simulink model "SrmUnlineSplineMat7a4b"  (R2014a)
settings: Solver=ode45  StartTime=0.0  StopTime=2  MaxStep=5e-5  RelTol=1e-3
InitFcn:
  | Res=1.5
  | L_0=0.001;
libraries: powerlib x26
settings Model: Creator=Administrator  LastModifiedBy=Think127
settings DataIOCC: SignalLoggingSaveFormat=ModelDataLogs
settings OptimizationCC: ExpressionDepthLimit=2147483647
settings DebuggingCC: UnderspecifiedInitializationDetection=Classic  FcnCallInpInsideContextMsg=UseLocalSettings  StateNameClashWarn=warning
settings GRTTargetCC: CombineOutputUpdateFcns=off  GRTInterface=on

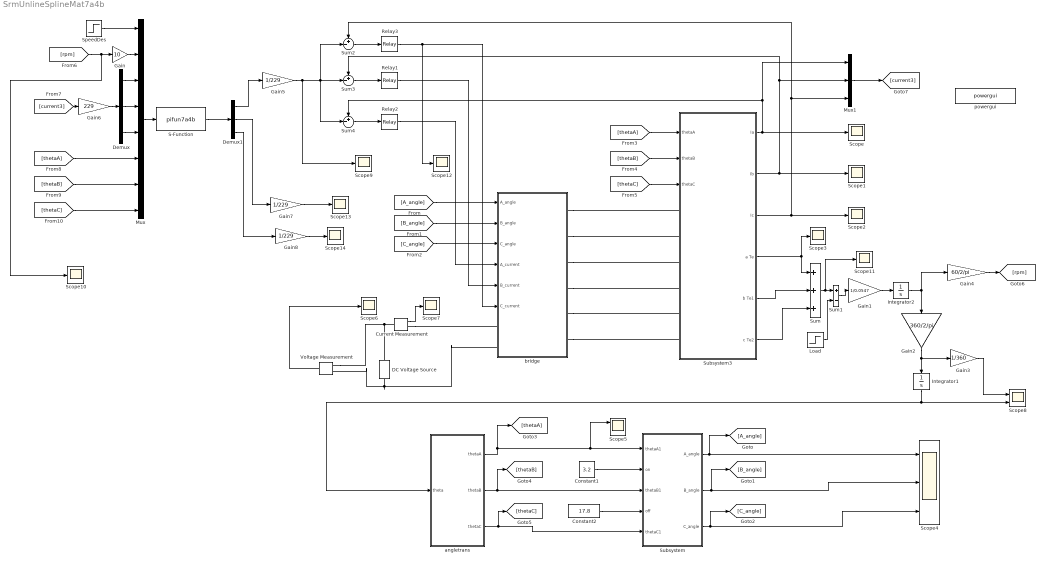
== system SrmUnlineSplineMat7a4b ==
  Constant1 : Constant  Value=3.2
  Constant2 : Constant  Value=17.8
  Current Measurement : powerlib/Measurements/Current Measurement  PhasorSimulation=off  OutputType=Complex  PSBequivalent=0
  DC Voltage Source : powerlib/Electrical Sources/DC Voltage Source  Amplitude=500  Measurements=None
  Demux : Demux  Outputs=3
  Demux1 : Demux  Outputs=3
  Gain : Gain  Gain=10
  Gain1 : Gain  Gain=1/0.0547
  Gain2 : Gain  Gain=360/2/pi
  Gain3 : Gain  Gain=1/360
  Gain4 : Gain  Gain=60/2/pi
  Gain5 : Gain  Gain=1/229
  Gain6 : Gain  Gain=229
  Gain7 : Gain  Gain=1/229
  Gain8 : Gain  Gain=1/229
  Integrator1 : Integrator  InitialCondition=6.5
  Integrator2 : Integrator
  Load : Step  Time=0.3  Before=10  After=10  SampleTime=0
  Mux : Mux  Inputs=8
  Mux1 : Mux  Inputs=3
  Relay1 : Relay  OnSwitchValue=0.1  OffSwitchValue=-0.001  OnOutputValue=0  OffOutputValue=1
  Relay2 : Relay  OnSwitchValue=0.1  OffSwitchValue=-0.001  OnOutputValue=0  OffOutputValue=1
  Relay3 : Relay  OnSwitchValue=0.1  OffSwitchValue=-0.001  OnOutputValue=0  OffOutputValue=1
  S-Function : S-Function  FunctionName=pifun7a4b  EnableBusSupport=off
  Scope{,1..3,6..7,9..14} (12 alike) : Scope
      Scope settings: TimeRange=2  YMin=0  YMax=2.75  SaveName=ScopeDataia
      Scope1 settings: TimeRange=0.01074006243496359  YMin=0  YMax=12.15970081836539
      Scope10 settings: TimeRange=2  YMin=599.75  YMax=600.5  SaveName=scopedataspeed  SampleInput=on  SampleTime=1/9600
      Scope11 settings: TimeRange=2  YMin=77.5  YMax=107.5  SaveName=ScopeData9te
      Scope12 settings: TimeRange=2  YMin=0.95  YMax=1.05  SaveName=ScopeData10
      Scope13 settings: TimeRange=2  YMin=11.9999999985  YMax=12.0000000015  SaveName=scopedataint  SampleInput=on  SampleTime=1/9600
      Scope14 settings: TimeRange=2  YMin=7.025  YMax=7.1  SaveName=scopedataintup  SampleInput=on  SampleTime=1/9600
      Scope2 settings: YMin=0  YMax=1.75  SaveName=ScopeData2
      Scope3 settings: TimeRange=2  YMin=-1.5  YMax=7  SaveName=ScopeData3
      Scope6 settings: YMin=39  YMax=41.5  SaveName=ScopeData8
      Scope7 settings: YMin=-1.75  YMax=2  SaveName=ScopeData12
      Scope9 settings: TimeRange=0.25  YMin=0  SaveName=ScopeData4
  Scope4 : Scope  NumInputPorts=3
      settings: TimeRange=0.0001268631901574406  YMin=0.95~-1~-1  YMax=1.05~1~1  SaveName=ScopeData5
  Scope5 : Scope  NumInputPorts=2
      settings: YMin=0~-1  YMax=45~1  SaveName=ScopeData7
  Scope8 : Scope  NumInputPorts=2
      settings: TimeRange=2  YMin=1.2~10  YMax=1.65~13.5  SaveName=ScopeData16_rpm_degree
  SpeedDes : Step  Time=0.3  Before=6000  After=8000  SampleTime=0
  Subsystem : Subsystem
  Subsystem3 : Subsystem
  Sum : Sum  Inputs=+++
  Sum1 : Sum  Inputs=+-
  Sum2 : Sum  Inputs=+-|
  Sum3 : Sum  Inputs=+-|
  Sum4 : Sum  Inputs=+-|
  Voltage Measurement : powerlib/Measurements/Voltage Measurement  PhasorSimulation=off  OutputType=Complex  PSBequivalent=0
  angletrans : Subsystem
  bridge : Subsystem
  powergui : powerlib/powergui  Priority=1  SimulationMode=Discrete  SolverType=Tustin  SampleTime=50e-6  frequency=60  SPID=off  DisableSnubberDevices=off  DisableRonSwitches=off  DisableVfSwitches=off  SwTol=0  Interpol=off  DisplayEquations=off  Ts=0  methode=off  frequencyindice=0  Pbase=100e6  ErrMax=1e-4  Iterations=50  UnitsV=kV  UnitsW=MW  FunctionMessages=off  echomessages=off  HookPort=off  EnableUseOfTLC=off  x0status=blocks  RestoreLinks=warning  ResistiveCurrentMeasurement=off  Frange=[0:2:500]  Ylog=off  Xlog=on  ShowGrid=off  save=off  variable=ZData  structure=0  ZoomFFT=on  StartTime=0.0  cycles=1  DisplayStyle=1  fundamental=60  FreqAxis=off  MaxFrequency=1000  frequencyindicesteady=1  RmsSteady=1  display=off
  wires:
  Constant1/1 -> Subsystem/2(on)
  Constant2/1 -> Subsystem/4(off)
  Subsystem3/1(Ia) -> Scope/1, Mux1/1, Sum4/1
  Subsystem3/3(Ic) -> Scope2/1, Mux1/3, Sum2/1
  Subsystem3/2(Ib) -> Scope1/1, Mux1/2, Sum3/1
  Voltage Measurement/1 -> Scope6/1
  Current Measurement/1 -> Scope7/1
  Subsystem3/4(a Te) -> Scope3/1, Sum/1
  Subsystem3/5(b Te1) -> Sum/2
  Subsystem3/6(c Te2) -> Sum/3
  Sum/1 -> Sum1/1, Scope11/1
  Gain1/1 -> Integrator2/1
  Integrator1/1 -> angletrans/1(theta), Scope8/2
  Integrator2/1 -> Gain4/1, Gain2/1
  Gain2/1 -> Integrator1/1, Gain3/1
  Relay2/1 -> bridge/4(A_current)
  Relay1/1 -> bridge/5(B_current)
  Relay3/1 -> Scope12/1, bridge/6(C_current)
  Gain3/1 -> Scope8/1
  Subsystem/1(A_angle) -> [A_angle], Scope4/1
  [A_angle] -> bridge/1(A_angle)
  Subsystem/2(B_angle) -> [B_angle], Scope4/2
  Subsystem/3(C_angle) -> [C_angle], Scope4/3
  [B_angle] -> bridge/2(B_angle)
  [C_angle] -> bridge/3(C_angle)
  angletrans/1(thetaA) -> Scope5/1, Subsystem/1(thetaA1), [thetaA]
  [thetaA] -> Subsystem3/1(thetaA)
  angletrans/2(thetaB) -> [thetaB], Subsystem/3(thetaB1)
  angletrans/3(thetaC) -> [thetaC], Subsystem/5(thetaC1)
  [thetaB] -> Subsystem3/2(thetaB)
  [thetaC] -> Subsystem3/3(thetaC)
  Load/1 -> Sum1/2
  Gain4/1 -> [rpm]
  [rpm] -> Scope10/1, Gain/1
  SpeedDes/1 -> Mux/1
  Sum2/1 -> Relay3/1
  Sum4/1 -> Relay2/1
  Sum3/1 -> Relay1/1
  Mux/1 -> S-Function/1
  Gain/1 -> Mux/2
  Gain5/1 -> Scope9/1, Sum2/2, Sum4/2, Sum3/2
  Mux1/1 -> [current3]
  Demux/1 -> Mux/3
  Demux/2 -> Mux/4
  Demux/3 -> Mux/5
  [current3] -> Gain6/1
  Gain6/1 -> Demux/1
  [thetaA] -> Mux/6
  [thetaB] -> Mux/7
  [thetaC] -> Mux/8
  S-Function/1 -> Demux1/1
  Demux1/1 -> Gain5/1
  Demux1/2 -> Gain7/1
  Demux1/3 -> Gain8/1
  Gain7/1 -> Scope13/1
  Gain8/1 -> Scope14/1
  Sum1/1 -> Gain1/1
  connections:
  DC Voltage Source/RConn1 -- Voltage Measurement/LConn1 -- Current Measurement/LConn1
  DC Voltage Source/LConn1 -- Voltage Measurement/LConn2 -- bridge/LConn2
  bridge/RConn2 -- Subsystem3/LConn2
  bridge/RConn4 -- Subsystem3/LConn4
  bridge/RConn6 -- Subsystem3/LConn6
  bridge/RConn5 -- Subsystem3/LConn5
  bridge/RConn3 -- Subsystem3/LConn3
  Current Measurement/RConn1 -- bridge/LConn1
  bridge/RConn1 -- Subsystem3/LConn1

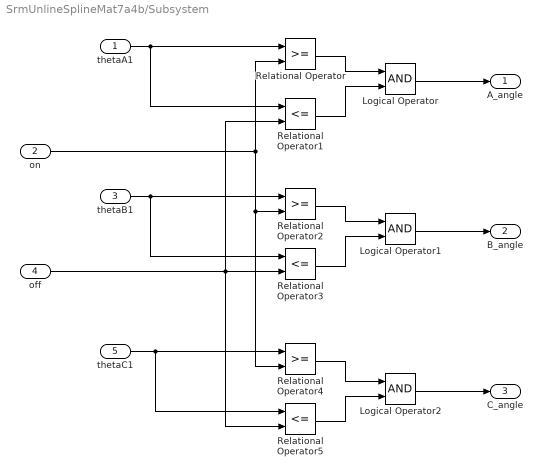
== system SrmUnlineSplineMat7a4b/Subsystem ==
  thetaA1 : Inport
  on : Inport  Port=2
  thetaB1 : Inport  Port=3
  off : Inport  Port=4
  thetaC1 : Inport  Port=5
  Logical Operator : Logic  AllPortsSameDT=off  OutDataTypeStr=boolean
  Logical Operator1 : Logic  AllPortsSameDT=off  OutDataTypeStr=boolean
  Logical Operator2 : Logic  AllPortsSameDT=off  OutDataTypeStr=boolean
  Relational Operator : RelationalOperator  OutDataTypeStr=boolean
  Relational Operator1 : RelationalOperator  Operator=<=  OutDataTypeStr=boolean
  Relational Operator2 : RelationalOperator  OutDataTypeStr=boolean
  Relational Operator3 : RelationalOperator  Operator=<=  OutDataTypeStr=boolean
  Relational Operator4 : RelationalOperator  OutDataTypeStr=boolean
  Relational Operator5 : RelationalOperator  Operator=<=  OutDataTypeStr=boolean
  A_angle : Outport
  B_angle : Outport  Port=2
  C_angle : Outport  Port=3
  wires:
  thetaA1/1 -> Relational Operator/1, Relational Operator1/1
  thetaB1/1 -> Relational Operator2/1, Relational Operator3/1
  thetaC1/1 -> Relational Operator4/1, Relational Operator5/1
  on/1 -> Relational Operator/2, Relational Operator2/2, Relational Operator4/2
  off/1 -> Relational Operator1/2, Relational Operator3/2, Relational Operator5/2
  Relational Operator/1 -> Logical Operator/1
  Relational Operator1/1 -> Logical Operator/2
  Relational Operator2/1 -> Logical Operator1/1
  Relational Operator3/1 -> Logical Operator1/2
  Relational Operator4/1 -> Logical Operator2/1
  Relational Operator5/1 -> Logical Operator2/2
  Logical Operator/1 -> A_angle/1
  Logical Operator1/1 -> B_angle/1
  Logical Operator2/1 -> C_angle/1

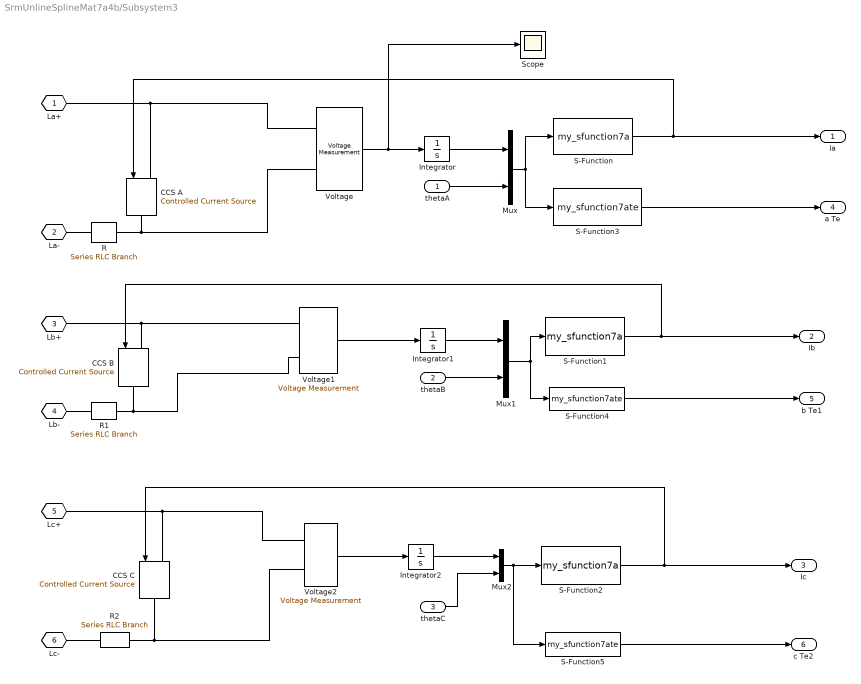
== system SrmUnlineSplineMat7a4b/Subsystem3 ==
  thetaA : Inport
  thetaB : Inport  Port=2
  thetaC : Inport  Port=3
  CCS A : powerlib/Electrical Sources/Controlled Current Source  Initialize=on  Source_Type=AC  Amplitude=0  Phase=0  Frequency=0  Measurements=None
  CCS B : powerlib/Electrical Sources/Controlled Current Source  Initialize=on  Source_Type=AC  Amplitude=0  Phase=0  Frequency=0  Measurements=None
  CCS C : powerlib/Electrical Sources/Controlled Current Source  Initialize=on  Source_Type=AC  Amplitude=0  Phase=0  Frequency=0  Measurements=None
  Integrator : Integrator  LimitOutput=on  LowerSaturationLimit=0
  Integrator1 : Integrator  LimitOutput=on  LowerSaturationLimit=0
  Integrator2 : Integrator  LimitOutput=on  LowerSaturationLimit=0
  Mux : Mux  Inputs=2
  Mux1 : Mux  Inputs=2
  Mux2 : Mux  Inputs=2
  R : powerlib/Elements/Series RLC Branch  LConnTagsString=__new0  RConnTagsString=__new0  BranchType=R  Resistance=Res  Inductance=L_0  SetiL0=off  InitialCurrent=0  Capacitance=1.0  Setx0=off  InitialVoltage=0  Measurements=None
  R1 : powerlib/Elements/Series RLC Branch  LConnTagsString=__new0  RConnTagsString=__new0  BranchType=R  Resistance=Res  Inductance=L_0  SetiL0=off  InitialCurrent=0  Capacitance=1.0  Setx0=off  InitialVoltage=0  Measurements=None
  R2 : powerlib/Elements/Series RLC Branch  LConnTagsString=__new0  RConnTagsString=__new0  BranchType=R  Resistance=Res  Inductance=L_0  SetiL0=off  InitialCurrent=0  Capacitance=1.0  Setx0=off  InitialVoltage=0  Measurements=None
  S-Function : S-Function  FunctionName=my_sfunction7a  EnableBusSupport=off
  S-Function1 : S-Function  FunctionName=my_sfunction7a  EnableBusSupport=off
  S-Function2 : S-Function  FunctionName=my_sfunction7a  EnableBusSupport=off
  S-Function3 : S-Function  FunctionName=my_sfunction7ate  EnableBusSupport=off
  S-Function4 : S-Function  FunctionName=my_sfunction7ate  EnableBusSupport=off
  S-Function5 : S-Function  FunctionName=my_sfunction7ate  EnableBusSupport=off
  Scope : Scope
      settings: TimeRange=2  YMin=-600  YMax=500  SaveName=ScopeData11
  Voltage : powerlib/Measurements/Voltage Measurement  PhasorSimulation=off  OutputType=Complex  PSBequivalent=0
  Voltage1 : powerlib/Measurements/Voltage Measurement  PhasorSimulation=off  OutputType=Complex  PSBequivalent=0
  Voltage2 : powerlib/Measurements/Voltage Measurement  PhasorSimulation=off  OutputType=Complex  PSBequivalent=0
  La+ : PMIOPort  Tag=PMCPort  Port=1  Side=Left
  La- : PMIOPort  Tag=PMCPort  Port=2  Side=Left
  Lb+ : PMIOPort  Tag=PMCPort  Port=3  Side=Left
  Lb- : PMIOPort  Tag=PMCPort  Port=4  Side=Left
  Lc+ : PMIOPort  Tag=PMCPort  Port=5  Side=Left
  Lc- : PMIOPort  Tag=PMCPort  Port=6  Side=Left
  Ia : Outport
  Ib : Outport  Port=2
  Ic : Outport  Port=3
  a Te : Outport  Port=4
  b Te1 : Outport  Port=5
  c Te2 : Outport  Port=6
  wires:
  Mux/1 -> S-Function/1, S-Function3/1
  Integrator/1 -> Mux/1
  thetaA/1 -> Mux/2
  Voltage/1 -> Scope/1, Integrator/1
  Mux1/1 -> S-Function1/1, S-Function4/1
  Integrator1/1 -> Mux1/1
  thetaB/1 -> Mux1/2
  S-Function1/1 -> Ib/1, CCS B/1
  Voltage1/1 -> Integrator1/1
  Mux2/1 -> S-Function5/1, S-Function2/1
  Integrator2/1 -> Mux2/1
  thetaC/1 -> Mux2/2
  S-Function2/1 -> Ic/1, CCS C/1
  Voltage2/1 -> Integrator2/1
  S-Function/1 -> CCS A/1, Ia/1
  S-Function3/1 -> a Te/1
  S-Function4/1 -> b Te1/1
  S-Function5/1 -> c Te2/1
  connections:
  La+/RConn1 -- Voltage/LConn1 -- CCS A/LConn1
  La-/RConn1 -- R/RConn1
  Lb+/RConn1 -- CCS B/LConn1 -- Voltage1/LConn1
  Lb-/RConn1 -- R1/RConn1
  CCS B/RConn1 -- Voltage1/LConn2 -- R1/LConn1
  Lc+/RConn1 -- Voltage2/LConn1 -- CCS C/LConn1
  Lc-/RConn1 -- R2/RConn1
  CCS C/RConn1 -- Voltage2/LConn2 -- R2/LConn1
  CCS A/RConn1 -- Voltage/LConn2 -- R/LConn1

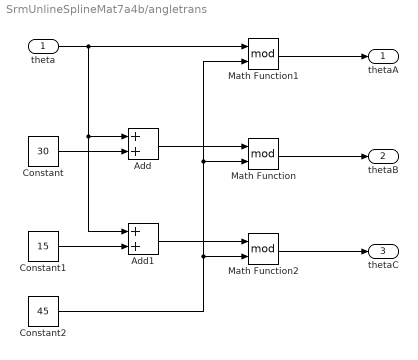
== system SrmUnlineSplineMat7a4b/angletrans ==
  theta : Inport
  Add : Sum
  Add1 : Sum
  Constant : Constant  Value=30
  Constant1 : Constant  Value=15
  Constant2 : Constant  Value=45
  Math Function : Math  Operator=mod  SaturateOnIntegerOverflow=on
  Math Function1 : Math  Operator=mod  SaturateOnIntegerOverflow=on
  Math Function2 : Math  Operator=mod  SaturateOnIntegerOverflow=on
  thetaA : Outport
  thetaB : Outport  Port=2
  thetaC : Outport  Port=3
  wires:
  Add1/1 -> Math Function2/1
  Add/1 -> Math Function/1
  theta/1 -> Math Function1/1, Add1/1, Add/1
  Constant/1 -> Add/2
  Constant1/1 -> Add1/2
  Constant2/1 -> Math Function2/2, Math Function/2, Math Function1/2
  Math Function2/1 -> thetaC/1
  Math Function/1 -> thetaB/1
  Math Function1/1 -> thetaA/1

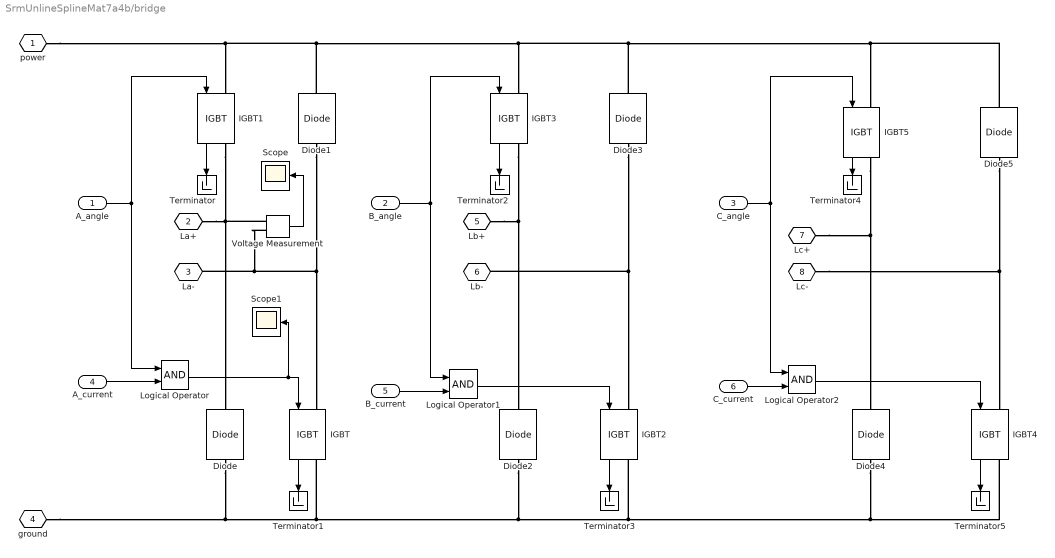
== system SrmUnlineSplineMat7a4b/bridge ==
  A_angle : Inport
  B_angle : Inport  Port=2
  C_angle : Inport  Port=3
  A_current : Inport  Port=4
  B_current : Inport  Port=5
  C_current : Inport  Port=6
  Diode{,1..5} (6 alike) : powerlib/Power Electronics/Diode  Ron=0.001  Lon=0  Vf=0.8  IC=0  UseSnubber=off  Rs=500  Cs=250e-9  Measurements=off
  IGBT{,1..5} (6 alike) : powerlib/Power Electronics/IGBT  Ron=0.001  Lon=0  Vf=1  Tf=1e-6  Tt=2e-6  IC=0  Rs=1e5  Cs=inf  Measurements=on
  Logical Operator : Logic  AllPortsSameDT=off  OutDataTypeStr=boolean
  Logical Operator1 : Logic  AllPortsSameDT=off  OutDataTypeStr=boolean
  Logical Operator2 : Logic  AllPortsSameDT=off  OutDataTypeStr=boolean
  Scope : Scope
      settings: YMin=-250  YMax=250  SaveName=ScopeData6
  Scope1 : Scope
      settings: YMin=57.14  YMax=57.2  SaveName=ScopeData13
  Terminator{,1..5} (6 alike) : Terminator
  Voltage Measurement : powerlib/Measurements/Voltage Measurement  PhasorSimulation=off  OutputType=Complex  PSBequivalent=0
  power : PMIOPort  Tag=PMCPort  Port=1  Side=Left
  La+ : PMIOPort  Tag=PMCPort  Port=2  Side=Right
  La- : PMIOPort  Tag=PMCPort  Port=3  Side=Right
  ground : PMIOPort  Tag=PMCPort  Port=4  Side=Left
  Lb+ : PMIOPort  Tag=PMCPort  Port=5  Side=Right
  Lb- : PMIOPort  Tag=PMCPort  Port=6  Side=Right
  Lc+ : PMIOPort  Tag=PMCPort  Port=7  Side=Right
  Lc- : PMIOPort  Tag=PMCPort  Port=8  Side=Right
  wires:
  IGBT4/1 -> Terminator5/1
  IGBT5/1 -> Terminator4/1
  C_angle/1 -> IGBT5/1, Logical Operator2/1
  IGBT2/1 -> Terminator3/1
  IGBT3/1 -> Terminator2/1
  B_angle/1 -> Logical Operator1/1, IGBT3/1
  IGBT/1 -> Terminator1/1
  IGBT1/1 -> Terminator/1
  A_angle/1 -> IGBT1/1, Logical Operator/1
  Voltage Measurement/1 -> Scope/1
  A_current/1 -> Logical Operator/2
  Logical Operator/1 -> Scope1/1, IGBT/1
  Logical Operator1/1 -> IGBT2/1
  B_current/1 -> Logical Operator1/2
  C_current/1 -> Logical Operator2/2
  Logical Operator2/1 -> IGBT4/1
  connections:
  Lc-/RConn1 -- IGBT4/LConn1 -- Diode5/LConn1
  Lc+/RConn1 -- IGBT5/RConn1 -- Diode4/RConn1
  Diode3/LConn1 -- IGBT2/LConn1 -- Lb-/RConn1
  Lb+/RConn1 -- IGBT3/RConn1 -- Diode2/RConn1
  Diode5/RConn1 -- Diode3/RConn1 -- Diode1/RConn1 -- power/RConn1 -- IGBT1/LConn1 -- IGBT3/LConn1 -- IGBT5/LConn1
  Diode1/LConn1 -- IGBT/LConn1 -- Voltage Measurement/LConn2 -- La-/RConn1
  La+/RConn1 -- Diode/RConn1 -- Voltage Measurement/LConn1 -- IGBT1/RConn1
  IGBT2/RConn1 -- ground/RConn1 -- Diode/LConn1 -- IGBT/RConn1 -- Diode2/LConn1 -- IGBT4/RConn1 -- Diode4/LConn1
